simulink model "bh_motor_and_full_mech_system"  (R2017a)
settings: Solver=ode15s  StartTime=0.0  StopTime=70  FixedStep=0.001  RelTol=1e-7  EnableMultiTasking=on
undefined symbols (not defined in the file or in its folder): g, Hz, L1x, L1y, L1z, mass1, sigbuilder_block, X, Y, Z
undefined symbols (not defined in the file): Ke
libraries: simulink_extras x18, nesl_utility x13, sm_lib x13, fl_lib x12, simulink x4, elec_lib x2, discretizing x1
settings Model: Creator=bhorton  LastModifiedBy=bhorton
settings SolverCC: ZeroCrossAlgorithm=Adaptive
settings OptimizationCC: LifeSpan=inf
settings DebuggingCC: SFUnexpectedBacktrackingDiag=warning  SFNoUnconditionalDefaultTransitionDiag=warning  SFExecutionAtInitializationDiag=none
settings GRTTargetCC: TargetLangStandard=C89/C90 (ANSI)
settings ConfigComp: CovMetricSettings=dw  CovHtmlReporting=on  CovSaveCumulativeToWorkspaceVar=on  CovSaveSingleToWorkspaceVar=on  CovExternalEMLEnable=off
settings SimscapeCC: SimscapeLogDataHistory=10000  SelectedTab=Simscape Multibody
settings ExplorerConfigSet: InternalSimMechanicsExplorerSettings="<ExplorerConfiguration><canonicalview>default</canonicalview><AnimationSetting><BasePlaybackSpeed>2</BasePlaybackSpeed><PlaybackSpeedFactor>1.0</PlaybackSpeedFactor></AnimationSetting><TilePanel><TileInfo><Tiles Columns=\"1\" Count=\"1\" Rows=\"1\"><Column Left=\"2\" Weight=\"1\"/><Column Left=\"820\"/><Row Top=\"2\" Weight=\"1\"/><Row Top=\"545\"/><Tile Height=\"1\" Width=\"1\" X=\"0\" Y=\"0\"/></Tiles></TileInfo><SceneInfo><SceneViewer><BGColor><R>0.60000002384185791</R><G>0.60000002384185791</G><B>0.60000002384185791</B></BGColor><Camera><DoPerspective>off</DoPerspective><Position><X>0.3018347345439823</X><Y>0.024415264242792611</Y><Z>0.21433472519445274</Z></Position><Center><X>0.024999999062628675</X><Y>0.30124999972414623</Y><Z>-0.062500010286905439</Z></Center><Up><X>-0.40824829046386751</X><Y>0.40824829046386751</Y><Z>0.81649658092772159</Z></Up><ViewLimDist>1</ViewLimDist><YLim>0.27384785473346712</YLim><XLim>0.4148743716842227</XLim></Camera></SceneViewer></SceneInfo></TilePanel><MechEditorPanel><Cameras/><GfxPanelCameraMap/></MechEditorPanel></ExplorerConfiguration>"

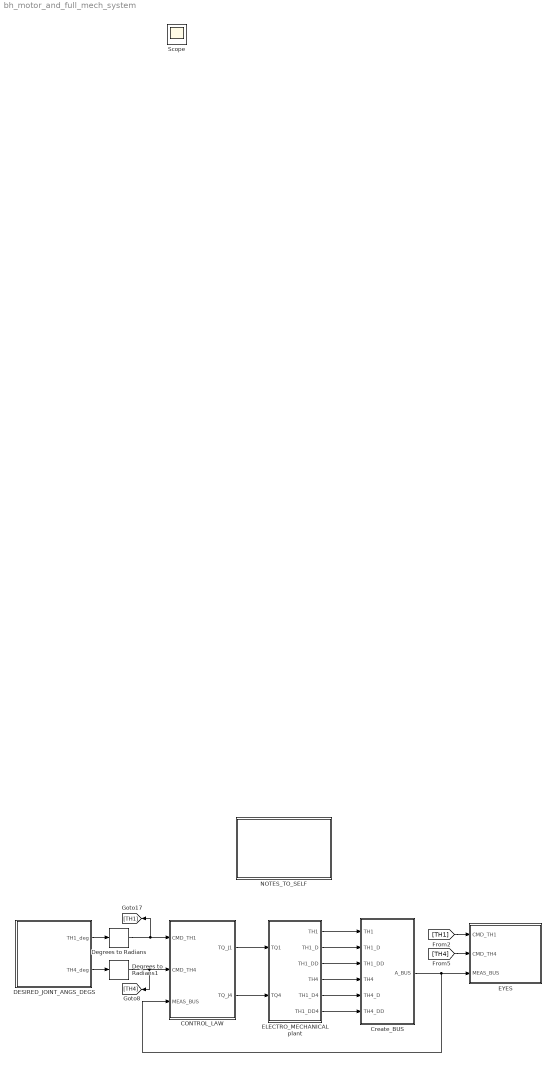
== system bh_motor_and_full_mech_system ==
  CONTROL_LAW : Subsystem
  Create_BUS : Subsystem
  DESIRED_JOINT_ANGS_DEGS : Subsystem  Tag=STV Subsys  LoadFcn=sigbuilder_block('load');  StartFcn=sigbuilder_block('start');  StopFcn=sigbuilder_block('stop');  ClipboardFcn=sigbuilder_block('clipboard');  mask(Sigbuilder block){tuvar=[0:10]}
      mask help: Simulink:masks:SigbuilderBlock_MD
      mask init:
      | if ~strcmp(get_param(bdroot(gcbh),'SimulationStatus'),'stopped') tuvar = sigbuilder_block('maskInit'); end
      settings: CopyFcn=sigbuilder_block('copy');  DeleteFcn=sigbuilder_block('delete');  ModelCloseFcn=sigbuilder_block('modelClose');  PreSaveFcn=sigbuilder_block('preSave');  PauseFcn=sigbuilder_block('pause');  ContinueFcn=sigbuilder_block('continue');  NameChangeFcn=sigbuilder_block('namechange');  OpenFcn=sigbuilder_block('open',[6 30 1428 681.75 ]);  CloseFcn=sigbuilder_block('close');
      mask Display: plot(0, 0, 100, 100,[2, 2, 32, 32, 2], [68, 8, 8, 68, 68],[32, 2], [38, 38], [32, 19, 2],[53, 60, 44], [32, 17, 17, 2],[16, 16, 31, 31]);txt = getActiveGroup(gcbh);text(2, 100, txt,'verticalAlignment', 'top');
  Degrees to Radians : simulink_extras/Transformations/Degrees to Radians
  Degrees to Radians1 : simulink_extras/Transformations/Degrees to Radians
  ELECTRO_MECHANICAL plant : Subsystem
  EYES : Subsystem
  NOTES_TO_SELF : Subsystem
  Scope : Scope
  wires:
  DESIRED_JOINT_ANGS_DEGS/1(TH1_deg) -> Degrees to Radians/1
  Degrees to Radians/1 -> CONTROL_LAW/1(CMD_TH1), [TH1]
  Degrees to Radians1/1 -> CONTROL_LAW/2(CMD_TH4), [TH4]
  DESIRED_JOINT_ANGS_DEGS/2(TH4_deg) -> Degrees to Radians1/1
  CONTROL_LAW/1(TQ_J1) -> ELECTRO_MECHANICAL plant/1(TQ1)
  CONTROL_LAW/2(TQ_J4) -> ELECTRO_MECHANICAL plant/2(TQ4)
  [TH4] -> EYES/2(CMD_TH4)
  Create_BUS/1(A_BUS) -> EYES/3(MEAS_BUS), CONTROL_LAW/3(MEAS_BUS)
  [TH1] -> EYES/1(CMD_TH1)
  ELECTRO_MECHANICAL plant/1(TH1) -> Create_BUS/1(TH1)
  ELECTRO_MECHANICAL plant/2(TH1_D) -> Create_BUS/2(TH1_D)
  ELECTRO_MECHANICAL plant/3(TH1_DD) -> Create_BUS/3(TH1_DD)
  ELECTRO_MECHANICAL plant/4(TH4) -> Create_BUS/4(TH4)
  ELECTRO_MECHANICAL plant/5(TH1_D4) -> Create_BUS/5(TH4_D)
  ELECTRO_MECHANICAL plant/6(TH1_DD4) -> Create_BUS/6(TH4_DD)

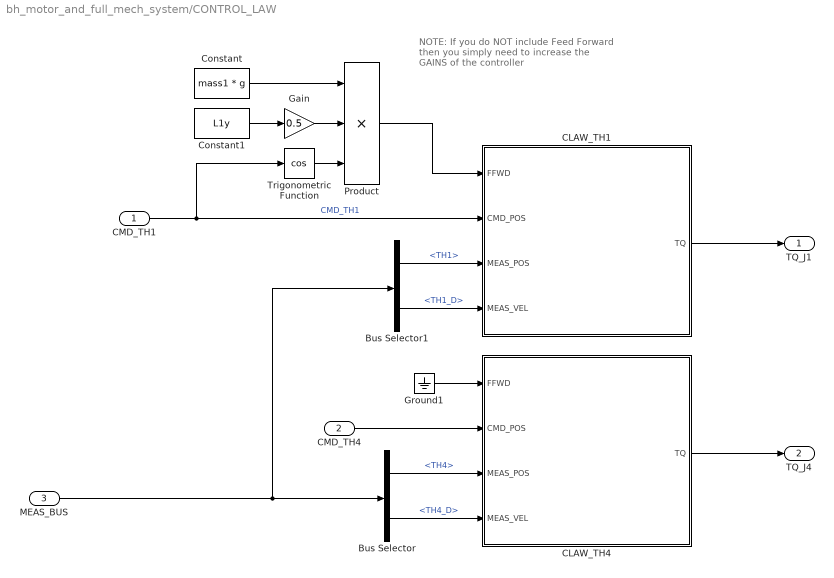
== system bh_motor_and_full_mech_system/CONTROL_LAW ==
  note: NOTE:
      | If you do NOT include Feed Forward
      | then you simply need to increase the GAINS of the controller
  CMD_TH1 : Inport
  CMD_TH4 : Inport  Port=2
  MEAS_BUS : Inport  Port=3
  Bus Selector : BusSelector  OutputSignals=TH4,TH4_D
  Bus Selector1 : BusSelector  OutputSignals=TH1,TH1_D
  CLAW_TH1 : Subsystem
  CLAW_TH4 : Subsystem
  Constant : Constant  Value=mass1 * g
  Constant1 : Constant  Value=L1y
  Gain : Gain  Gain=0.5
  Ground1 : Ground
  Product : Product  Inputs=3
  Trigonometric Function : Trigonometry  Operator=cos
  TQ_J1 : Outport
  TQ_J4 : Outport  Port=2
  wires:
  MEAS_BUS/1 -> Bus Selector1/1, Bus Selector/1
  CMD_TH4/1 -> CLAW_TH4/2(CMD_POS)
  Bus Selector/2 -> CLAW_TH4/4(MEAS_VEL)  "<TH4_D>"
  Bus Selector/1 -> CLAW_TH4/3(MEAS_POS)  "<TH4>"
  Bus Selector1/1 -> CLAW_TH1/3(MEAS_POS)  "<TH1>"
  Bus Selector1/2 -> CLAW_TH1/4(MEAS_VEL)  "<TH1_D>"
  Ground1/1 -> CLAW_TH4/1(FFWD)
  CMD_TH1/1 -> CLAW_TH1/2(CMD_POS), Trigonometric Function/1  "CMD_TH1"
  Constant/1 -> Product/1
  Constant1/1 -> Gain/1
  Product/1 -> CLAW_TH1/1(FFWD)
  Gain/1 -> Product/2
  Trigonometric Function/1 -> Product/3
  CLAW_TH1/1(TQ) -> TQ_J1/1
  CLAW_TH4/1(TQ) -> TQ_J4/1

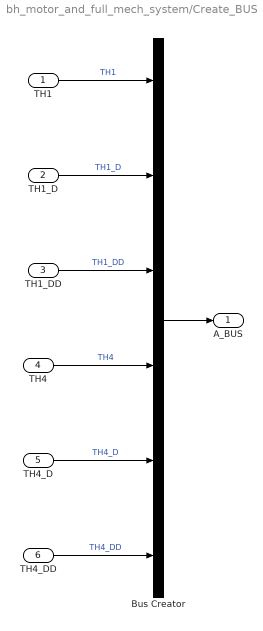
== system bh_motor_and_full_mech_system/Create_BUS ==
  TH1 : Inport
  TH1_D : Inport  Port=2
  TH1_DD : Inport  Port=3
  TH4 : Inport  Port=4
  TH4_D : Inport  Port=5
  TH4_DD : Inport  Port=6
  Bus Creator : BusCreator  Inputs=6
  A_BUS : Outport
  wires:
  TH1_DD/1 -> Bus Creator/3  "TH1_DD"
  TH1_D/1 -> Bus Creator/2  "TH1_D"
  TH1/1 -> Bus Creator/1  "TH1"
  Bus Creator/1 -> A_BUS/1
  TH4_DD/1 -> Bus Creator/6  "TH4_DD"
  TH4_D/1 -> Bus Creator/5  "TH4_D"
  TH4/1 -> Bus Creator/4  "TH4"

== system bh_motor_and_full_mech_system/DESIRED_JOINT_ANGS_DEGS ==
  Demux : Demux  Tag=STV Demux  Outputs=2
  FromWs : FromWorkspace  Tag=STV FromWs  VariableName=tuvar  SampleTime=0
      SigBuilderData=|
      | common.afterFinalStr = 'Extrapolate'
      | common.sampleTime = 0
      | dataSet(1).timeRange = [0 60]
      | dataSet(1).name = 'SCENARIO_A_JUST_TH1'
      | dataSet(2).timeRange = [0 60]
      | dataSet(2).name = 'SCENARIO_B_JUST_TH4'
      | dataSet(3).timeRange = [0 60]
      | dataSet(3).name = 'SCENARIO_C_TH1_and_TH4'
      | dataSet(4).timeRange = [0 60]
      | dataSet(4).name = 'SCENARIO_D_TH1_and_TH4'
      | dataSet(5).timeRange = [0 70]
      | dataSet(5).name = 'SCENARIO_E'
      | sbobj.Groups(1).Name = 'SCENARIO_A_JUST_TH1'
      | sbobj.Groups(1).Signals(1).Name = 'TH1_deg'
      | sbobj.Groups(1).Signals(1).XData = [0 20 20 60]
      | sbobj.Groups(1).Signals(1).YData = [0 0 45 45]
      | sbobj.Groups(1).Signals(2).Name = 'TH4_deg'
      | sbobj.Groups(1).Signals(2).XData = [0 60]
      | sbobj.Groups(1).Signals(2).YData = [0 0]
      | sbobj.Groups(1).TimeRange = [0 60]
      | sbobj.Groups(2).Name = 'SCENARIO_B_JUST_TH4'
      | sbobj.Groups(2).Signals(1).Name = 'TH1_deg'
      | sbobj.Groups(2).Signals(1).XData = [0 20 60]
      | sbobj.Groups(2).Signals(1).YData = [0 0 0]
      | sbobj.Groups(2).Signals(2).Name = 'TH4_deg'
      | sbobj.Groups(2).Signals(2).XData = [0 20 20 60]
      | sbobj.Groups(2).Signals(2).YData = [0 0 45 45]
      | sbobj.Groups(2).TimeRange = [0 60]
      | sbobj.Groups(3).Name = 'SCENARIO_C_TH1_and_TH4'
      | sbobj.Groups(3).Signals(1).Name = 'TH1_deg'
      | sbobj.Groups(3).Signals(1).XData = [0 10 10 40 60]
      | sbobj.Groups(3).Signals(1).YData = [0 0 45 45 0]
      | sbobj.Groups(3).Signals(2).Name = 'TH4_deg'
      | sbobj.Groups(3).Signals(2).XData = [0 14.95 14.95 30 60]
      | sbobj.Groups(3).Signals(2).YData = [0 0 45 45 0]
      | sbobj.Groups(3).TimeRange = [0 60]
      | sbobj.Groups(4).Name = 'SCENARIO_D_TH1_and_TH4'
      | sbobj.Groups(4).Signals(1).Name = 'TH1_deg'
      | sbobj.Groups(4).Signals(1).XData = [0 10 40 60]
      | sbobj.Groups(4).Signals(1).YData = [0 45 45 0]
      | sbobj.Groups(4).Signals(2).Name = 'TH4_deg'
      | sbobj.Groups(4).Signals(2).XData = [0 10 30 60]
      | sbobj.Groups(4).Signals(2).YData = [0 45 45 0]
      | sbobj.Groups(4).TimeRange = [0 60]
      | sbobj.Groups(5).Name = 'SCENARIO_E'
      | sbobj.Groups(5).Signals(1).Name = 'TH1_deg'
      | sbobj.Groups(5).Signals(1).XData = [0 35.15 45.4 60 70]
      | sbobj.Groups(5).Signals(1).YData = [0 0 45 -45 0]
      | sbobj.Groups(5).Signals(2).Name = 'TH4_deg'
      | sbobj.Groups(5).Signals(2).XData = [0 10 25 30 70]
      | sbobj.Groups(5).Signals(2).YData = [0 -90 90 0 0]
      | sbobj.Groups(5).TimeRange = [0 70]
  TH1_deg : Outport  Tag=STV Outport
  TH4_deg : Outport  Tag=STV Outport  Port=2
  wires:
  FromWs/1 -> Demux/1
  Demux/1 -> TH1_deg/1
  Demux/2 -> TH4_deg/1

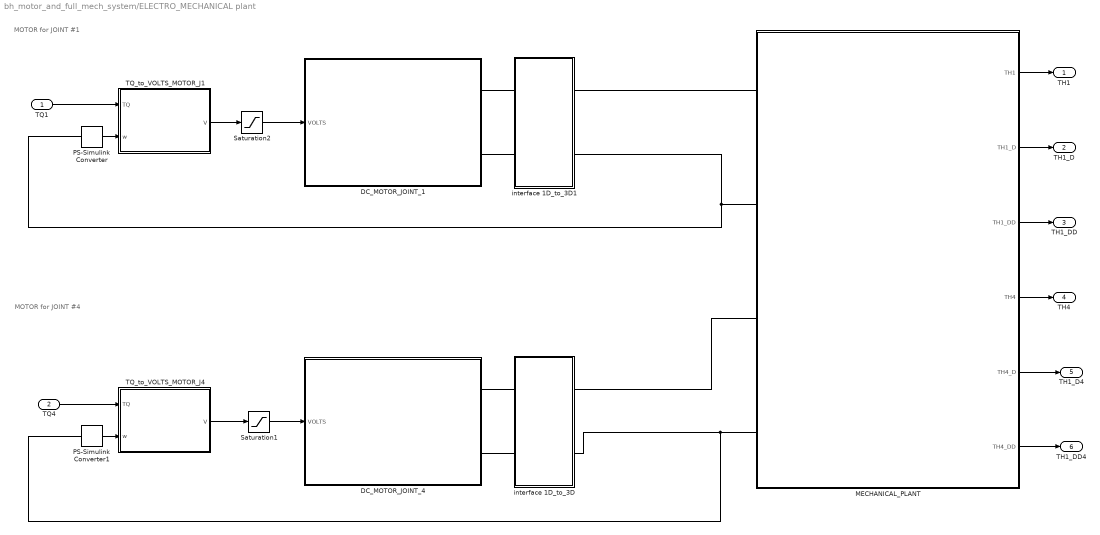
== system bh_motor_and_full_mech_system/ELECTRO_MECHANICAL plant ==
  note: MOTOR for JOINT #4
  note: MOTOR for JOINT #1
  TQ1 : Inport
  TQ4 : Inport  Port=2
  DC_MOTOR_JOINT_1 : Subsystem
      mask Display: image('bh_PIC_MOTOR.jpg');
  DC_MOTOR_JOINT_4 : Subsystem
      mask Display: image('bh_PIC_MOTOR.jpg');
  MECHANICAL_PLANT : Subsystem  VariantControl=Variant1
  PS-Simulink Converter : nesl_utility/PS-Simulink Converter  PhysicalDomain=network_engine_domain  SubClassName=ps_output  LeftPortType=input  RightPortType=output  PseudoPeriodic=off  Frequencies=[]  Unit=rad/s  AffineConversion=off
      settings: AttributesFormatString=Units = %<Unit>
  PS-Simulink Converter1 : nesl_utility/PS-Simulink Converter  PhysicalDomain=network_engine_domain  SubClassName=ps_output  LeftPortType=input  RightPortType=output  PseudoPeriodic=off  Frequencies=[]  Unit=rad/s  AffineConversion=off
      settings: AttributesFormatString=Units = %<Unit>
  Saturation1 : Saturate  UpperLimit=12  LowerLimit=-12
      settings: AttributesFormatString=|
      | Vmax = %<UpperLimit>
      | Vmin = %<LowerLimit>
  Saturation2 : Saturate  UpperLimit=12  LowerLimit=-12
      settings: AttributesFormatString=|
      | Vmax = %<UpperLimit>
      | Vmin = %<LowerLimit>
  TQ_to_VOLTS_MOTOR_J1 : Subsystem  mask(DC motor (w_IN and TQ_out)){R=5.0117, K=0.57296 *0.875, Kb=Ke, b=8.20705e-3}
      mask prompts: R "Armature resistance (ohms)"; K "Torque constant (N.m/A)"; Kb "Back Emf constant (V.sec/rad)"; b "damping value (N.m.sec/rad)"
      mask help: A DC motor model that outputs required VOLTAGE needed to deliver a specified TORQUE
      mask DialogControl Control2 Prompt: NOTE:  with SI units, the Toque constant (Ka) and Back EMF constant(Kb) are the same.
      mask DialogControl Container9 Prompt: Electrical
      mask Display: fprintf('DC motor\n(TQ_IN \n and \n V_out)');
  TQ_to_VOLTS_MOTOR_J4 : Subsystem  mask(DC motor (w_IN and TQ_out)){R=5.0117, K=0.57296 *0.875, Kb=Ke, b=8.20705e-3}
      mask prompts: R "Armature resistance (ohms)"; K "Torque constant (N.m/A)"; Kb "Back Emf constant (V.sec/rad)"; b "damping value (N.m.sec/rad)"
      mask help: A DC motor model that outputs required VOLTAGE needed to deliver a specified TORQUE
      mask DialogControl Control2 Prompt: NOTE:  with SI units, the Toque constant (Ka) and Back EMF constant(Kb) are the same.
      mask DialogControl Container9 Prompt: Electrical
      mask Display: fprintf('DC motor\n(TQ_IN \n and \n V_out)');
  interface 1D_to_3D : Subsystem
  interface 1D_to_3D1 : Subsystem
  TH1 : Outport
  TH1_D : Outport  Port=2
  TH1_DD : Outport  Port=3
  TH4 : Outport  Port=4
  TH1_D4 : Outport  Port=5
  TH1_DD4 : Outport  Port=6
  wires:
  TQ_to_VOLTS_MOTOR_J1/1(V) -> Saturation2/1
  PS-Simulink Converter/1 -> TQ_to_VOLTS_MOTOR_J1/2(w)
  TQ1/1 -> TQ_to_VOLTS_MOTOR_J1/1(TQ)
  PS-Simulink Converter1/1 -> TQ_to_VOLTS_MOTOR_J4/2(w)
  TQ4/1 -> TQ_to_VOLTS_MOTOR_J4/1(TQ)
  TQ_to_VOLTS_MOTOR_J4/1(V) -> Saturation1/1
  MECHANICAL_PLANT/1(TH1) -> TH1/1
  MECHANICAL_PLANT/2(TH1_D) -> TH1_D/1
  MECHANICAL_PLANT/3(TH1_DD) -> TH1_DD/1
  MECHANICAL_PLANT/4(TH4) -> TH4/1
  MECHANICAL_PLANT/5(TH4_D) -> TH1_D4/1
  MECHANICAL_PLANT/6(TH4_DD) -> TH1_DD4/1
  Saturation1/1 -> DC_MOTOR_JOINT_4/1(VOLTS)
  Saturation2/1 -> DC_MOTOR_JOINT_1/1(VOLTS)
  connections:
  interface 1D_to_3D/RConn1 -- MECHANICAL_PLANT/LConn3
  PS-Simulink Converter/LConn1 -- interface 1D_to_3D1/RConn2 -- MECHANICAL_PLANT/LConn2
  interface 1D_to_3D/RConn2 -- PS-Simulink Converter1/LConn1 -- MECHANICAL_PLANT/LConn4
  MECHANICAL_PLANT/LConn1 -- interface 1D_to_3D1/RConn1
  interface 1D_to_3D/LConn1 -- DC_MOTOR_JOINT_4/RConn1
  interface 1D_to_3D/LConn2 -- DC_MOTOR_JOINT_4/RConn2
  interface 1D_to_3D1/LConn1 -- DC_MOTOR_JOINT_1/RConn1
  interface 1D_to_3D1/LConn2 -- DC_MOTOR_JOINT_1/RConn2

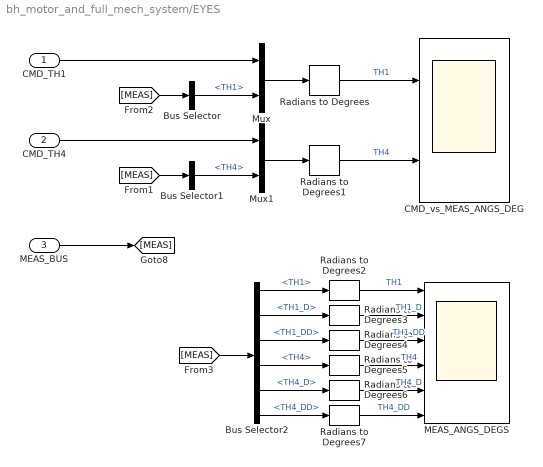
== system bh_motor_and_full_mech_system/EYES ==
  CMD_TH1 : Inport
  CMD_TH4 : Inport  Port=2
  MEAS_BUS : Inport  Port=3
  Bus Selector : BusSelector  OutputSignals=TH1
  Bus Selector1 : BusSelector  OutputSignals=TH4
  Bus Selector2 : BusSelector  OutputSignals=TH1,TH1_D,TH1_DD,TH4,TH4_D,TH4_DD
  CMD_vs_MEAS_ANGS_DEG : Scope  NumInputPorts=2
  MEAS_ANGS_DEGS : Scope  NumInputPorts=6
  Mux : Mux  Inputs=2
  Mux1 : Mux  Inputs=2
  Radians to Degrees{,1..7} (8 alike) : simulink_extras/Transformations/Radians to Degrees
  wires:
  MEAS_BUS/1 -> [MEAS]
  CMD_TH1/1 -> Mux/1
  Bus Selector/1 -> Mux/2  "<TH1>"
  [MEAS] -> Bus Selector/1
  Mux/1 -> Radians to Degrees/1
  CMD_TH4/1 -> Mux1/1
  Bus Selector1/1 -> Mux1/2  "<TH4>"
  [MEAS] -> Bus Selector1/1
  Mux1/1 -> Radians to Degrees1/1
  Radians to Degrees1/1 -> CMD_vs_MEAS_ANGS_DEG/2  "TH4"
  Radians to Degrees/1 -> CMD_vs_MEAS_ANGS_DEG/1  "TH1"
  [MEAS] -> Bus Selector2/1
  Bus Selector2/6 -> Radians to Degrees7/1  "<TH4_DD>"
  Bus Selector2/3 -> Radians to Degrees4/1  "<TH1_DD>"
  Bus Selector2/4 -> Radians to Degrees5/1  "<TH4>"
  Bus Selector2/5 -> Radians to Degrees6/1  "<TH4_D>"
  Bus Selector2/2 -> Radians to Degrees3/1  "<TH1_D>"
  Bus Selector2/1 -> Radians to Degrees2/1  "<TH1>"
  Radians to Degrees2/1 -> MEAS_ANGS_DEGS/1  "TH1"
  Radians to Degrees3/1 -> MEAS_ANGS_DEGS/2  "TH1_D"
  Radians to Degrees4/1 -> MEAS_ANGS_DEGS/3  "TH1_DD"
  Radians to Degrees5/1 -> MEAS_ANGS_DEGS/4  "TH4"
  Radians to Degrees6/1 -> MEAS_ANGS_DEGS/5  "TH4_D"
  Radians to Degrees7/1 -> MEAS_ANGS_DEGS/6  "TH4_DD"

== system bh_motor_and_full_mech_system/NOTES_TO_SELF ==
  note: NOTES to self:
      | Had to enable these:

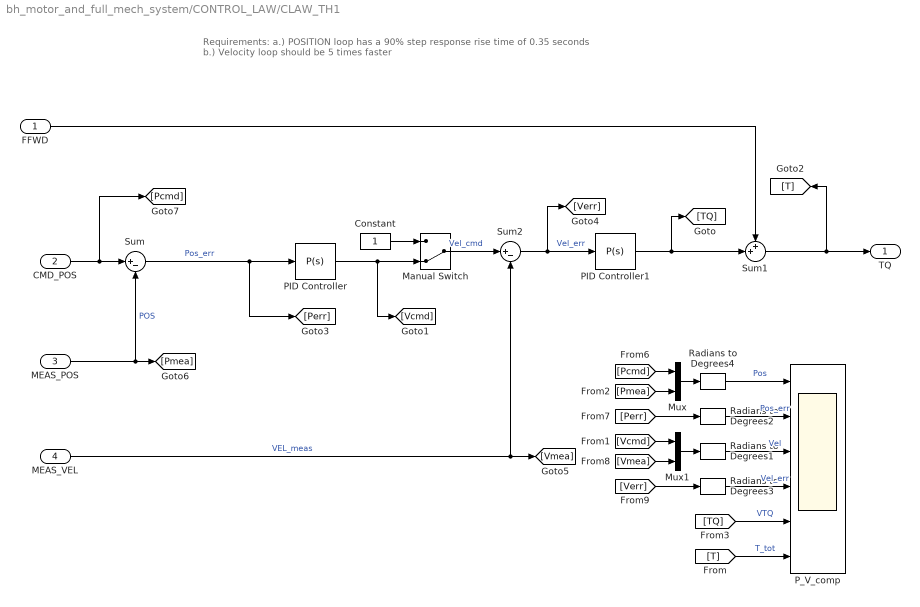
== system bh_motor_and_full_mech_system/CONTROL_LAW/CLAW_TH1 ==
  note: Requirements:
      | a.) POSITION loop has a 90% step response
      | rise time of 0.35 seconds
      |
      | b.) Velocity loop should be 5 times faster
  FFWD : Inport
  CMD_POS : Inport  Port=2
  MEAS_POS : Inport  Port=3
  MEAS_VEL : Inport  Port=4
  Constant : Constant
  Manual Switch : ManualSwitch  CurrentSetting=0
  Mux : Mux  Inputs=2
  Mux1 : Mux  Inputs=2
  PID Controller : simulink/Continuous/PID Controller  Controller=P  TimeDomain=Continuous-time  SampleTime=-1  IntegratorMethod=Forward Euler  FilterMethod=Forward Euler  Form=Parallel  UseFilter=on  ControllerParametersSource=internal  P=5.58549433794614  I=0  D=0  N=100  InitialConditionSource=internal  InitialConditionForIntegrator=0  InitialConditionForFilter=0  ExternalReset=none  LimitOutput=off  UpperSaturationLimit=inf  LowerSaturationLimit=-inf  LinearizeAsGain=on  AntiWindupMode=none  Kb=1  TrackingMode=off  Kt=1  PParamMin=[]  PParamMax=[]  IParamMin=[]  IParamMax=[]  DParamMin=[]  DParamMax=[]  NParamMin=[]  NParamMax=[]  KbParamMin=[]  KbParamMax=[]  KtParamMin=[]  KtParamMax=[]  POutMin=[]  POutMax=[]  IOutMin=[]  IOutMax=[]  DOutMin=[]  DOutMax=[]  NOutMin=[]  NOutMax=[]  KbOutMin=[]  KbOutMax=[]  KtOutMin=[]  KtOutMax=[]  IntegratorOutMin=[]  IntegratorOutMax=[]  FilterOutMin=[]  FilterOutMax=[]  SumOutMin=[]  SumOutMax=[]  SumI1OutMin=[]  SumI1OutMax=[]  SumI2OutMin=[]  SumI2OutMax=[]  SumI3OutMin=[]  SumI3OutMax=[]  SumDOutMin=[]  SumDOutMax=[]  SaturationOutMin=[]  SaturationOutMax=[]  IntegratorContinuousStateAttributes=''  IntegratorStateMustResolveToSignalObject=off  IntegratorRTWStateStorageClass=Auto  FilterContinuousStateAttributes=''  FilterStateMustResolveToSignalObject=off  FilterRTWStateStorageClass=Auto  DifferentiatorICPrevScaledInput=0  DifferentiatorOutMin=[]  DifferentiatorOutMax=[]  InitialConditionSetting=State (most efficient)
  PID Controller1 : simulink/Continuous/PID Controller  Controller=P  TimeDomain=Continuous-time  SampleTime=-1  IntegratorMethod=Forward Euler  FilterMethod=Forward Euler  Form=Parallel  UseFilter=on  ControllerParametersSource=internal  P=1  I=1  D=0  N=100  InitialConditionSource=internal  InitialConditionForIntegrator=0  InitialConditionForFilter=0  ExternalReset=none  LimitOutput=off  UpperSaturationLimit=inf  LowerSaturationLimit=-inf  LinearizeAsGain=on  AntiWindupMode=none  Kb=1  TrackingMode=off  Kt=1  PParamMin=[]  PParamMax=[]  IParamMin=[]  IParamMax=[]  DParamMin=[]  DParamMax=[]  NParamMin=[]  NParamMax=[]  KbParamMin=[]  KbParamMax=[]  KtParamMin=[]  KtParamMax=[]  POutMin=[]  POutMax=[]  IOutMin=[]  IOutMax=[]  DOutMin=[]  DOutMax=[]  NOutMin=[]  NOutMax=[]  KbOutMin=[]  KbOutMax=[]  KtOutMin=[]  KtOutMax=[]  IntegratorOutMin=[]  IntegratorOutMax=[]  FilterOutMin=[]  FilterOutMax=[]  SumOutMin=[]  SumOutMax=[]  SumI1OutMin=[]  SumI1OutMax=[]  SumI2OutMin=[]  SumI2OutMax=[]  SumI3OutMin=[]  SumI3OutMax=[]  SumDOutMin=[]  SumDOutMax=[]  SaturationOutMin=[]  SaturationOutMax=[]  IntegratorContinuousStateAttributes=''  IntegratorStateMustResolveToSignalObject=off  IntegratorRTWStateStorageClass=Auto  FilterContinuousStateAttributes=''  FilterStateMustResolveToSignalObject=off  FilterRTWStateStorageClass=Auto  DifferentiatorICPrevScaledInput=0  DifferentiatorOutMin=[]  DifferentiatorOutMax=[]  InitialConditionSetting=State (most efficient)
  P_V_comp : Scope  NumInputPorts=6
  Radians to Degrees{1..4} (4 alike) : simulink_extras/Transformations/Radians to Degrees
  Sum : Sum  Inputs=|+-
  Sum1 : Sum  Inputs=++|
  Sum2 : Sum  Inputs=|+-
  TQ : Outport
  wires:
  FFWD/1 -> Sum1/1
  CMD_POS/1 -> [Pcmd], Sum/1
  MEAS_VEL/1 -> [Vmea], Sum2/2  "VEL_meas"
  MEAS_POS/1 -> [Pmea], Sum/2  "POS"
  Sum2/1 -> PID Controller1/1, [Verr]  "Vel_err"
  Manual Switch/1 -> Sum2/1  "Vel_cmd"
  Constant/1 -> Manual Switch/1
  Sum/1 -> PID Controller/1, [Perr]  "Pos_err"
  PID Controller/1 -> Manual Switch/2, [Vcmd]
  Sum1/1 -> TQ/1, [T]
  Mux/1 -> Radians to Degrees4/1
  [Pcmd] -> Mux/1
  [Pmea] -> Mux/2
  Mux1/1 -> Radians to Degrees1/1
  [Vcmd] -> Mux1/1
  [Vmea] -> Mux1/2
  [Verr] -> Radians to Degrees3/1
  [Perr] -> Radians to Degrees2/1
  Radians to Degrees3/1 -> P_V_comp/4  "Vel_err"
  Radians to Degrees2/1 -> P_V_comp/2  "Pos_err"
  Radians to Degrees1/1 -> P_V_comp/3  "Vel"
  Radians to Degrees4/1 -> P_V_comp/1  "Pos"
  [TQ] -> P_V_comp/5  "VTQ"
  [T] -> P_V_comp/6  "T_tot"
  PID Controller1/1 -> Sum1/2, [TQ]

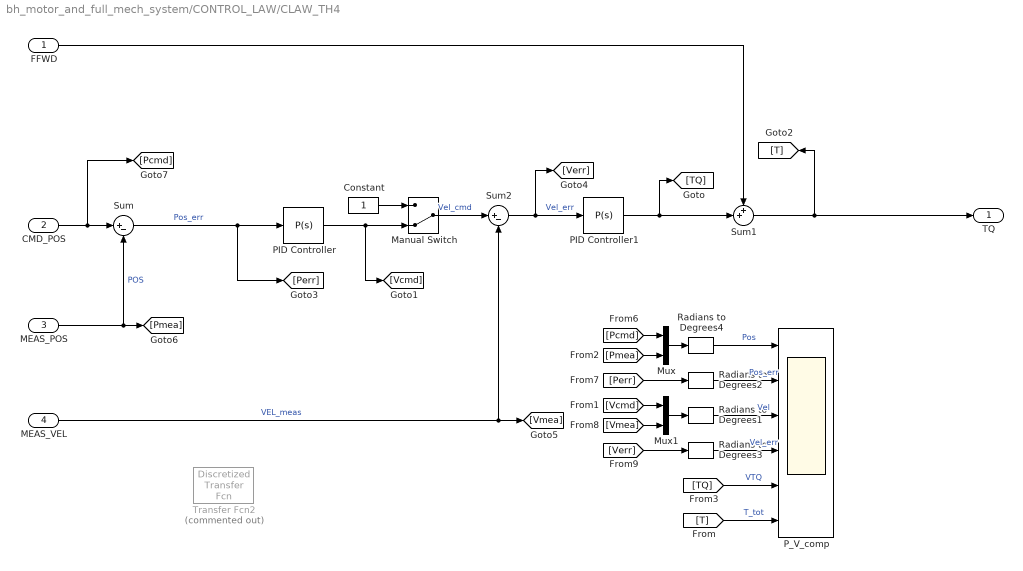
== system bh_motor_and_full_mech_system/CONTROL_LAW/CLAW_TH4 ==
  FFWD : Inport
  CMD_POS : Inport  Port=2
  MEAS_POS : Inport  Port=3
  MEAS_VEL : Inport  Port=4
  Constant : Constant
  Manual Switch : ManualSwitch  CurrentSetting=0
  Mux : Mux  Inputs=2
  Mux1 : Mux  Inputs=2
  PID Controller : simulink/Continuous/PID Controller  Controller=P  TimeDomain=Continuous-time  SampleTime=-1  IntegratorMethod=Forward Euler  FilterMethod=Forward Euler  Form=Parallel  UseFilter=on  ControllerParametersSource=internal  P=5.58549433794614  I=1  D=0  N=100  InitialConditionSource=internal  InitialConditionForIntegrator=0  InitialConditionForFilter=0  ExternalReset=none  LimitOutput=off  UpperSaturationLimit=inf  LowerSaturationLimit=-inf  LinearizeAsGain=on  AntiWindupMode=none  Kb=1  TrackingMode=off  Kt=1  PParamMin=[]  PParamMax=[]  IParamMin=[]  IParamMax=[]  DParamMin=[]  DParamMax=[]  NParamMin=[]  NParamMax=[]  KbParamMin=[]  KbParamMax=[]  KtParamMin=[]  KtParamMax=[]  POutMin=[]  POutMax=[]  IOutMin=[]  IOutMax=[]  DOutMin=[]  DOutMax=[]  NOutMin=[]  NOutMax=[]  KbOutMin=[]  KbOutMax=[]  KtOutMin=[]  KtOutMax=[]  IntegratorOutMin=[]  IntegratorOutMax=[]  FilterOutMin=[]  FilterOutMax=[]  SumOutMin=[]  SumOutMax=[]  SumI1OutMin=[]  SumI1OutMax=[]  SumI2OutMin=[]  SumI2OutMax=[]  SumI3OutMin=[]  SumI3OutMax=[]  SumDOutMin=[]  SumDOutMax=[]  SaturationOutMin=[]  SaturationOutMax=[]  IntegratorContinuousStateAttributes=''  IntegratorStateMustResolveToSignalObject=off  IntegratorRTWStateStorageClass=Auto  FilterContinuousStateAttributes=''  FilterStateMustResolveToSignalObject=off  FilterRTWStateStorageClass=Auto  DifferentiatorICPrevScaledInput=0  DifferentiatorOutMin=[]  DifferentiatorOutMax=[]  InitialConditionSetting=State (most efficient)
  PID Controller1 : simulink/Continuous/PID Controller  Controller=P  TimeDomain=Continuous-time  SampleTime=-1  IntegratorMethod=Forward Euler  FilterMethod=Forward Euler  Form=Parallel  UseFilter=on  ControllerParametersSource=internal  P=1  I=1  D=0  N=100  InitialConditionSource=internal  InitialConditionForIntegrator=0  InitialConditionForFilter=0  ExternalReset=none  LimitOutput=off  UpperSaturationLimit=inf  LowerSaturationLimit=-inf  LinearizeAsGain=on  AntiWindupMode=none  Kb=1  TrackingMode=off  Kt=1  PParamMin=[]  PParamMax=[]  IParamMin=[]  IParamMax=[]  DParamMin=[]  DParamMax=[]  NParamMin=[]  NParamMax=[]  KbParamMin=[]  KbParamMax=[]  KtParamMin=[]  KtParamMax=[]  POutMin=[]  POutMax=[]  IOutMin=[]  IOutMax=[]  DOutMin=[]  DOutMax=[]  NOutMin=[]  NOutMax=[]  KbOutMin=[]  KbOutMax=[]  KtOutMin=[]  KtOutMax=[]  IntegratorOutMin=[]  IntegratorOutMax=[]  FilterOutMin=[]  FilterOutMax=[]  SumOutMin=[]  SumOutMax=[]  SumI1OutMin=[]  SumI1OutMax=[]  SumI2OutMin=[]  SumI2OutMax=[]  SumI3OutMin=[]  SumI3OutMax=[]  SumDOutMin=[]  SumDOutMax=[]  SaturationOutMin=[]  SaturationOutMax=[]  IntegratorContinuousStateAttributes=''  IntegratorStateMustResolveToSignalObject=off  IntegratorRTWStateStorageClass=Auto  FilterContinuousStateAttributes=''  FilterStateMustResolveToSignalObject=off  FilterRTWStateStorageClass=Auto  DifferentiatorICPrevScaledInput=0  DifferentiatorOutMin=[]  DifferentiatorOutMax=[]  InitialConditionSetting=State (most efficient)
  P_V_comp : Scope  NumInputPorts=6
  Radians to Degrees{1..4} (4 alike) : simulink_extras/Transformations/Radians to Degrees
  Sum : Sum  Inputs=|+-
  Sum1 : Sum  Inputs=++|
  Sum2 : Sum  Inputs=|+-
  Transfer Fcn2 : discretizing/Discretized Transfer Fcn  Commented=on  Numerator=[100]  Denominator=[1 100]  AbsTol=auto  SampleTime=0.001  method=tustin  Wc=1
  TQ : Outport
  wires:
  FFWD/1 -> Sum1/1
  CMD_POS/1 -> [Pcmd], Sum/1
  MEAS_VEL/1 -> [Vmea], Sum2/2  "VEL_meas"
  MEAS_POS/1 -> [Pmea], Sum/2  "POS"
  Sum2/1 -> PID Controller1/1, [Verr]  "Vel_err"
  Manual Switch/1 -> Sum2/1  "Vel_cmd"
  Constant/1 -> Manual Switch/1
  Sum/1 -> PID Controller/1, [Perr]  "Pos_err"
  PID Controller/1 -> Manual Switch/2, [Vcmd]
  Sum1/1 -> TQ/1, [T]
  Mux/1 -> Radians to Degrees4/1
  [Pcmd] -> Mux/1
  [Pmea] -> Mux/2
  Mux1/1 -> Radians to Degrees1/1
  [Vcmd] -> Mux1/1
  [Vmea] -> Mux1/2
  [Verr] -> Radians to Degrees3/1
  [Perr] -> Radians to Degrees2/1
  Radians to Degrees3/1 -> P_V_comp/4  "Vel_err"
  Radians to Degrees2/1 -> P_V_comp/2  "Pos_err"
  Radians to Degrees1/1 -> P_V_comp/3  "Vel"
  Radians to Degrees4/1 -> P_V_comp/1  "Pos"
  [TQ] -> P_V_comp/5  "VTQ"
  [T] -> P_V_comp/6  "T_tot"
  PID Controller1/1 -> Sum1/2, [TQ]

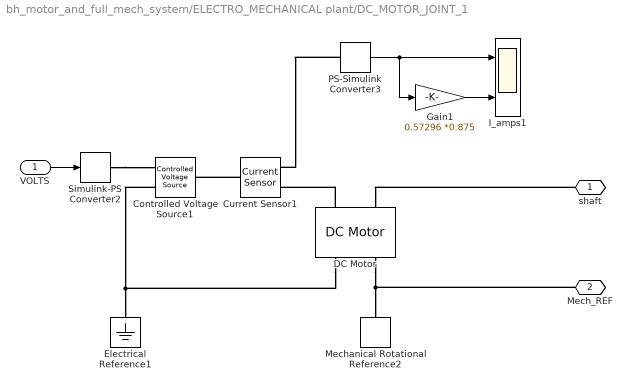
== system bh_motor_and_full_mech_system/ELECTRO_MECHANICAL plant/DC_MOTOR_JOINT_1 ==
  VOLTS : Inport
  Controlled Voltage Source1 : fl_lib/Electrical/Electrical Sources/Controlled Voltage Source
  Current Sensor1 : fl_lib/Electrical/Electrical Sensors/Current Sensor
  DC Motor : elec_lib/Actuators & Drivers/Rotational Actuators/DC Motor  parameterization=2  Ra=2 Ohm  La=1e-4 H  emf_or_torque=2  Kv=7.2e-5 V/rpm  Ki=0.0083 N*m/A  T_stall=1.2 N*m  w_max=200 rpm  w_rated=1.5e+4 rpm  P_rated=0.08 W  V_rated=12 V  J=4.5e-5 kg*m^2  lam_param=2  lam=0.7e-5 N*m/(rad/s)  i_noload=300 mA  V_i_noload=12 V  speed0=0 rpm  alpha=0.00393 1/K  Tmeas=25 C  thermal_mass=100 J/K  initial_temperature=25 C
  Electrical Reference1 : fl_lib/Electrical/Electrical Elements/Electrical Reference
  Gain1 : Gain  Gain=0.57296 *0.875
  I_amps1 : Scope  NumInputPorts=2
  Mechanical Rotational Reference2 : fl_lib/Mechanical/Rotational Elements/Mechanical Rotational Reference
  PS-Simulink Converter3 : nesl_utility/PS-Simulink Converter  PhysicalDomain=network_engine_domain  SubClassName=ps_output  LeftPortType=input  RightPortType=output  PseudoPeriodic=off  Frequencies=[]  Unit=A  AffineConversion=off
  Simulink-PS Converter2 : nesl_utility/Simulink-PS Converter  PhysicalDomain=network_engine_domain  SubClassName=ps_input  LeftPortType=input  RightPortType=output  PseudoPeriodic=off  Frequencies=[]  NoiseDistribution=none  NoiseParameters=[]  Unit=V  AffineConversion=off  FilteringAndDerivatives=filter  SimscapeFilterOrder=1  InputFilterTimeConstant=0.001  UdotUserProvided=1
  shaft : PMIOPort  Port=1  Side=Right
  Mech_REF : PMIOPort  Port=2  Side=Right
  wires:
  Gain1/1 -> I_amps1/2
  VOLTS/1 -> Simulink-PS Converter2/1
  PS-Simulink Converter3/1 -> Gain1/1, I_amps1/1
  connections:
  DC Motor/LConn1 -- Current Sensor1/RConn2
  DC Motor/RConn2 -- Mechanical Rotational Reference2/LConn1 -- Mech_REF/RConn1
  Current Sensor1/LConn1 -- Controlled Voltage Source1/LConn1
  Simulink-PS Converter2/RConn1 -- Controlled Voltage Source1/RConn1
  shaft/RConn1 -- DC Motor/LConn2
  Controlled Voltage Source1/RConn2 -- DC Motor/RConn1 -- Electrical Reference1/LConn1
  PS-Simulink Converter3/LConn1 -- Current Sensor1/RConn1

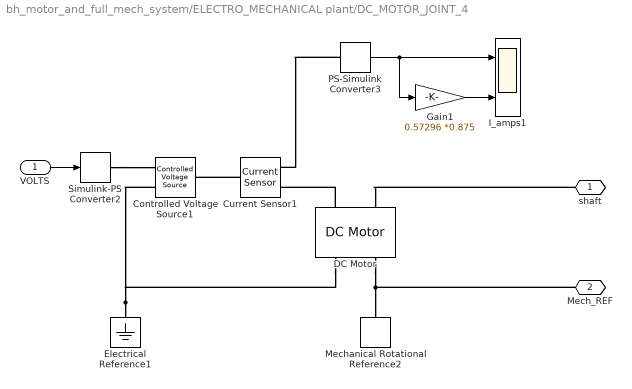
== system bh_motor_and_full_mech_system/ELECTRO_MECHANICAL plant/DC_MOTOR_JOINT_4 ==
  VOLTS : Inport
  Controlled Voltage Source1 : fl_lib/Electrical/Electrical Sources/Controlled Voltage Source
  Current Sensor1 : fl_lib/Electrical/Electrical Sensors/Current Sensor
  DC Motor : elec_lib/Actuators & Drivers/Rotational Actuators/DC Motor  parameterization=2  Ra=2 Ohm  La=1e-4 H  emf_or_torque=2  Kv=7.2e-5 V/rpm  Ki=0.0083 N*m/A  T_stall=1.2 N*m  w_max=200 rpm  w_rated=1.5e+4 rpm  P_rated=0.08 W  V_rated=12 V  J=4.5e-5 kg*m^2  lam_param=2  lam=0.7e-5 N*m/(rad/s)  i_noload=300 mA  V_i_noload=12 V  speed0=0 rpm  alpha=0.00393 1/K  Tmeas=25 C  thermal_mass=100 J/K  initial_temperature=25 C
  Electrical Reference1 : fl_lib/Electrical/Electrical Elements/Electrical Reference
  Gain1 : Gain  Gain=0.57296 *0.875
  I_amps1 : Scope  NumInputPorts=2
  Mechanical Rotational Reference2 : fl_lib/Mechanical/Rotational Elements/Mechanical Rotational Reference
  PS-Simulink Converter3 : nesl_utility/PS-Simulink Converter  PhysicalDomain=network_engine_domain  SubClassName=ps_output  LeftPortType=input  RightPortType=output  PseudoPeriodic=off  Frequencies=[]  Unit=A  AffineConversion=off
  Simulink-PS Converter2 : nesl_utility/Simulink-PS Converter  PhysicalDomain=network_engine_domain  SubClassName=ps_input  LeftPortType=input  RightPortType=output  PseudoPeriodic=off  Frequencies=[]  NoiseDistribution=none  NoiseParameters=[]  Unit=V  AffineConversion=off  FilteringAndDerivatives=filter  SimscapeFilterOrder=1  InputFilterTimeConstant=0.001  UdotUserProvided=1
  shaft : PMIOPort  Port=1  Side=Right
  Mech_REF : PMIOPort  Port=2  Side=Right
  wires:
  Gain1/1 -> I_amps1/2
  VOLTS/1 -> Simulink-PS Converter2/1
  PS-Simulink Converter3/1 -> Gain1/1, I_amps1/1
  connections:
  DC Motor/LConn1 -- Current Sensor1/RConn2
  DC Motor/RConn2 -- Mech_REF/RConn1 -- Mechanical Rotational Reference2/LConn1
  Current Sensor1/LConn1 -- Controlled Voltage Source1/LConn1
  Simulink-PS Converter2/RConn1 -- Controlled Voltage Source1/RConn1
  shaft/RConn1 -- DC Motor/LConn2
  Electrical Reference1/LConn1 -- Controlled Voltage Source1/RConn2 -- DC Motor/RConn1
  PS-Simulink Converter3/LConn1 -- Current Sensor1/RConn1

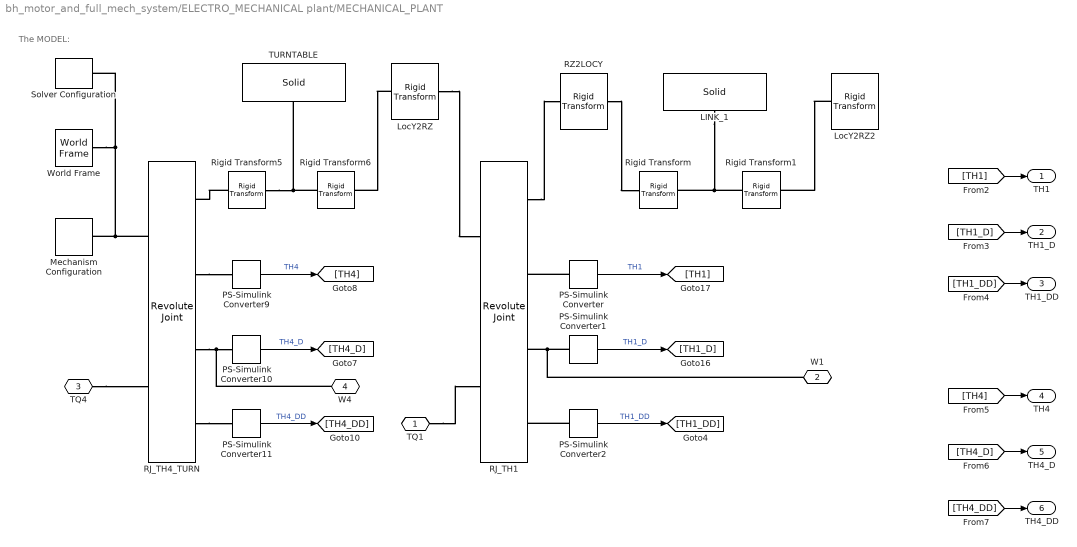
== system bh_motor_and_full_mech_system/ELECTRO_MECHANICAL plant/MECHANICAL_PLANT ==
  note: The MODEL:
  LINK_1 : sm_lib/Body Elements/Solid  InertiaType=CalculateFromGeometry  Mass=1  MassUnits=kg  CenterOfMass=[0 0 0]  CenterOfMassUnits=m  MomentsOfInertia=[1 1 1]  MomentsOfInertiaUnits=kg*m^2  ProductsOfInertia=[0 0 0]  ProductsOfInertiaUnits=kg*m^2  DensityBased=on  Density=density  DensityUnits=kg/(m^3)  DoExposeReferenceFrame=on  SerializedFrames=<Frames/>  GraphicType=FromGeometry  MarkerShape=Sphere  MarkerSize=10  GraphicVisPropType=SimpleVisualProperties  GraphicDiffuseColor=[0.2 0.2 1.0]  GraphicSpecularColor=[0.5 0.5 0.5 1.0]  GraphicAmbientColor=[0.15 0.15 0.15 1.0]  GraphicEmissiveColor=[0.0 0.0 0.0 1.0]  GraphicShininess=75  GraphicOpacity=1.0  GeometryShape=Brick  RectangleSize=[1 1]  RectangleSizeUnits=m  BrickDimensions=[L1x, L1y, L1z ]  BrickDimensionUnits=m  CylinderRadius=1  CylinderRadiusUnits=m  CylinderLength=1  CylinderLengthUnits=m  SphereRadius=1  SphereRadiusUnits=m  EllipsoidRadii=[1 1 1]  EllipsoidRadiiUnits=m  ExtrusionCrossSection=[1 1; -1 1; -1 -1; 1 -1]  ExtrusionCrossSectionUnits=m  ExtrusionLength=1  ExtrusionLengthUnits=m  PolygonNumSides=3  PolygonOuterRadius=1  PolygonOuterRadiusUnits=m  ExtGeomFileType=STEP  ExtGeomFileUnits=m  RevolutionCrossSection=[1 1; 1 -1; 2 -1; 2 1]  RevolutionCrossSectionUnits=m  RevolutionExtent=Full  RevolutionAngle=180  RevolutionAngleUnits=deg
  LocY2RZ : sm_lib/Frames and Transforms/Rigid Transform  TranslationMethod=None  TranslationStandardOffset=Hz/2  TranslationLengthUnit=m  TranslationStandardAxis=+Z  TranslationCartesianOffset=[0 0 0]  TranslationROffset=0  TranslationROffsetUnits=m  TranslationZOffset=0  TranslationZOffsetUnits=m  TranslationThetaOffset=0  TranslationThetaOffsetUnits=deg  RotationMethod=AlignedAxes  RotationAngleUnits=deg  RotationStandardAxis=+Z  RotationAngle=0.0  RotationArbitraryAxis=[0 0 1]  FollAlignAxisA=+X  BaseAlignAxisA=+Y  FollAlignAxisB=+Y  BaseAlignAxisB=+Z  RotationSequenceAxes=FollowerAxes  RotationSequence=XYX  RotationSequenceAngles=[0 0 0]  RotationSequenceAnglesUnits=deg  RotationMatrix=[1 0 0; 0 1 0; 0 0 1]
  LocY2RZ2 : sm_lib/Frames and Transforms/Rigid Transform  TranslationMethod=None  TranslationStandardOffset=Hz/2  TranslationLengthUnit=m  TranslationStandardAxis=+Z  TranslationCartesianOffset=[0 0 0]  TranslationROffset=0  TranslationROffsetUnits=m  TranslationZOffset=0  TranslationZOffsetUnits=m  TranslationThetaOffset=0  TranslationThetaOffsetUnits=deg  RotationMethod=AlignedAxes  RotationAngleUnits=deg  RotationStandardAxis=+Z  RotationAngle=0.0  RotationArbitraryAxis=[0 0 1]  FollAlignAxisA=+X  BaseAlignAxisA=+Y  FollAlignAxisB=+Y  BaseAlignAxisB=+Z  RotationSequenceAxes=FollowerAxes  RotationSequence=XYX  RotationSequenceAngles=[0 0 0]  RotationSequenceAnglesUnits=deg  RotationMatrix=[1 0 0; 0 1 0; 0 0 1]
  Mechanism Configuration : sm_lib/Utilities/Mechanism Configuration  UniformGravity=Constant  GravityVector=[0 0 -g ]  GravityUnits=m/s^2  LinearizationDelta=1e-4
  PS-Simulink Converter : nesl_utility/PS-Simulink Converter  PhysicalDomain=network_engine_domain  SubClassName=ps_output  LeftPortType=input  RightPortType=output  PseudoPeriodic=off  Frequencies=[]  Unit=rad  AffineConversion=off
  PS-Simulink Converter1 : nesl_utility/PS-Simulink Converter  PhysicalDomain=network_engine_domain  SubClassName=ps_output  LeftPortType=input  RightPortType=output  PseudoPeriodic=off  Frequencies=[]  Unit=rad/s  AffineConversion=off
  PS-Simulink Converter10 : nesl_utility/PS-Simulink Converter  PhysicalDomain=network_engine_domain  SubClassName=ps_output  LeftPortType=input  RightPortType=output  PseudoPeriodic=off  Frequencies=[]  Unit=rad/s  AffineConversion=off
  PS-Simulink Converter11 : nesl_utility/PS-Simulink Converter  PhysicalDomain=network_engine_domain  SubClassName=ps_output  LeftPortType=input  RightPortType=output  PseudoPeriodic=off  Frequencies=[]  Unit=rad/s^2  AffineConversion=off
  PS-Simulink Converter2 : nesl_utility/PS-Simulink Converter  PhysicalDomain=network_engine_domain  SubClassName=ps_output  LeftPortType=input  RightPortType=output  PseudoPeriodic=off  Frequencies=[]  Unit=rad/s^2  AffineConversion=off
  PS-Simulink Converter9 : nesl_utility/PS-Simulink Converter  PhysicalDomain=network_engine_domain  SubClassName=ps_output  LeftPortType=input  RightPortType=output  PseudoPeriodic=off  Frequencies=[]  Unit=rad  AffineConversion=off
  RJ_TH1 : sm_lib/Joints/Revolute Joint  SenseConstraintForce=off  SenseConstraintForceX=off  SenseConstraintForceY=off  SenseConstraintForceZ=off  SenseConstraintTorque=off  SenseConstraintTorqueX=off  SenseConstraintTorqueY=off  SenseConstraintTorqueZ=off  SenseTotalForce=off  SenseTotalForceX=off  SenseTotalForceY=off  SenseTotalForceZ=off  SenseTotalTorque=off  SenseTotalTorqueX=off  SenseTotalTorqueY=off  SenseTotalTorqueZ=off  CompositeWrenchDir=BaseOnFollower  CompositeWrenchFrame=BaseFrame  EquilibriumPosition=0  EquilibriumPositionUnits=deg  SpringStiffness=0  SpringStiffnessUnits=N*m/deg  DampingCoefficient=b1_damp  DampingCoefficientUnits=N*m/(rad/s)  TorqueActuationMode=InputTorque  MotionActuationMode=ComputedMotion  SensePosition=on  SenseVelocity=on  SenseAcceleration=on  SenseTorqueForce=off  PositionTargetSpecify=on  PositionTargetPriority=Low  PositionTargetValue=theta1_0  PositionTargetValueUnits=rad  VelocityTargetSpecify=on  VelocityTargetPriority=High  VelocityTargetValue=theta1_dot_0  VelocityTargetValueUnits=rad/s
      settings: AttributesFormatString=|
      | %<DampingCoefficient>
      | %<PositionTargetValue>
      | %<VelocityTargetValue>
  RJ_TH4_TURN : sm_lib/Joints/Revolute Joint  SenseConstraintForce=off  SenseConstraintForceX=off  SenseConstraintForceY=off  SenseConstraintForceZ=off  SenseConstraintTorque=off  SenseConstraintTorqueX=off  SenseConstraintTorqueY=off  SenseConstraintTorqueZ=off  SenseTotalForce=off  SenseTotalForceX=off  SenseTotalForceY=off  SenseTotalForceZ=off  SenseTotalTorque=off  SenseTotalTorqueX=off  SenseTotalTorqueY=off  SenseTotalTorqueZ=off  CompositeWrenchDir=BaseOnFollower  CompositeWrenchFrame=BaseFrame  EquilibriumPosition=0  EquilibriumPositionUnits=deg  SpringStiffness=0  SpringStiffnessUnits=N*m/deg  DampingCoefficient=b4_damp  DampingCoefficientUnits=N*m/(rad/s)  TorqueActuationMode=InputTorque  MotionActuationMode=ComputedMotion  SensePosition=on  SenseVelocity=on  SenseAcceleration=on  SenseTorqueForce=off  PositionTargetSpecify=on  PositionTargetPriority=Low  PositionTargetValue=theta4_0  PositionTargetValueUnits=rad  VelocityTargetSpecify=on  VelocityTargetPriority=High  VelocityTargetValue=theta4_dot_0  VelocityTargetValueUnits=rad/s
      settings: AttributesFormatString=|
      | %<DampingCoefficient>
      | %<PositionTargetValue>
      | %<VelocityTargetValue>
  RZ2LOCY : sm_lib/Frames and Transforms/Rigid Transform  TranslationMethod=None  TranslationStandardOffset=Hz/2  TranslationLengthUnit=m  TranslationStandardAxis=+Z  TranslationCartesianOffset=[0 0 0]  TranslationROffset=0  TranslationROffsetUnits=m  TranslationZOffset=0  TranslationZOffsetUnits=m  TranslationThetaOffset=0  TranslationThetaOffsetUnits=deg  RotationMethod=AlignedAxes  RotationAngleUnits=deg  RotationStandardAxis=+Z  RotationAngle=0.0  RotationArbitraryAxis=[0 0 1]  FollAlignAxisA=+Y  BaseAlignAxisA=+X  FollAlignAxisB=+X  BaseAlignAxisB=+Z  RotationSequenceAxes=FollowerAxes  RotationSequence=XYX  RotationSequenceAngles=[0 0 0]  RotationSequenceAnglesUnits=deg  RotationMatrix=[1 0 0; 0 1 0; 0 0 1]
  Rigid Transform : sm_lib/Frames and Transforms/Rigid Transform  TranslationMethod=StandardAxis  TranslationStandardOffset=L1y/2  TranslationLengthUnit=m  TranslationStandardAxis=+Y  TranslationCartesianOffset=[0 0 0]  TranslationROffset=0  TranslationROffsetUnits=m  TranslationZOffset=0  TranslationZOffsetUnits=m  TranslationThetaOffset=0  TranslationThetaOffsetUnits=deg  RotationMethod=None  RotationAngleUnits=deg  RotationStandardAxis=+Z  RotationAngle=0.0  RotationArbitraryAxis=[0 0 1]  FollAlignAxisA=+X  BaseAlignAxisA=+Y  FollAlignAxisB=+Y  BaseAlignAxisB=+Z  RotationSequenceAxes=FollowerAxes  RotationSequence=XYX  RotationSequenceAngles=[0 0 0]  RotationSequenceAnglesUnits=deg  RotationMatrix=[1 0 0; 0 1 0; 0 0 1]
  Rigid Transform1 : sm_lib/Frames and Transforms/Rigid Transform  TranslationMethod=StandardAxis  TranslationStandardOffset=L1y/2  TranslationLengthUnit=m  TranslationStandardAxis=+Y  TranslationCartesianOffset=[0 0 0]  TranslationROffset=0  TranslationROffsetUnits=m  TranslationZOffset=0  TranslationZOffsetUnits=m  TranslationThetaOffset=0  TranslationThetaOffsetUnits=deg  RotationMethod=None  RotationAngleUnits=deg  RotationStandardAxis=+Z  RotationAngle=0.0  RotationArbitraryAxis=[0 0 1]  FollAlignAxisA=+X  BaseAlignAxisA=+Y  FollAlignAxisB=+Y  BaseAlignAxisB=+Z  RotationSequenceAxes=FollowerAxes  RotationSequence=XYX  RotationSequenceAngles=[0 0 0]  RotationSequenceAnglesUnits=deg  RotationMatrix=[1 0 0; 0 1 0; 0 0 1]
  Rigid Transform5 : sm_lib/Frames and Transforms/Rigid Transform  TranslationMethod=StandardAxis  TranslationStandardOffset=Hz/2  TranslationLengthUnit=m  TranslationStandardAxis=-Z  TranslationCartesianOffset=[0 0 0]  TranslationROffset=0  TranslationROffsetUnits=m  TranslationZOffset=0  TranslationZOffsetUnits=m  TranslationThetaOffset=0  TranslationThetaOffsetUnits=deg  RotationMethod=None  RotationAngleUnits=deg  RotationStandardAxis=+Z  RotationAngle=0.0  RotationArbitraryAxis=[0 0 1]  FollAlignAxisA=+X  BaseAlignAxisA=+Y  FollAlignAxisB=+Y  BaseAlignAxisB=+Z  RotationSequenceAxes=FollowerAxes  RotationSequence=XYX  RotationSequenceAngles=[0 0 0]  RotationSequenceAnglesUnits=deg  RotationMatrix=[1 0 0; 0 1 0; 0 0 1]
  Rigid Transform6 : sm_lib/Frames and Transforms/Rigid Transform  TranslationMethod=StandardAxis  TranslationStandardOffset=Hz/2  TranslationLengthUnit=m  TranslationStandardAxis=+Z  TranslationCartesianOffset=[0 0 0]  TranslationROffset=0  TranslationROffsetUnits=m  TranslationZOffset=0  TranslationZOffsetUnits=m  TranslationThetaOffset=0  TranslationThetaOffsetUnits=deg  RotationMethod=None  RotationAngleUnits=deg  RotationStandardAxis=+Z  RotationAngle=0.0  RotationArbitraryAxis=[0 0 1]  FollAlignAxisA=+X  BaseAlignAxisA=+Y  FollAlignAxisB=+Y  BaseAlignAxisB=+Z  RotationSequenceAxes=FollowerAxes  RotationSequence=XYX  RotationSequenceAngles=[0 0 0]  RotationSequenceAnglesUnits=deg  RotationMatrix=[1 0 0; 0 1 0; 0 0 1]
  Solver Configuration : nesl_utility/Solver Configuration  PhysicalDomain=network_engine_domain  SubClassName=solver  LeftPortType=input  RightPortType=generic  Accelerate=off  Tones=[]  Harmonics=[]  SimulateNoise=off  Profile=off  UseLocalSampling=off  EnableSwitchedLinearOptims=on  FrequencyDomain=off  UseCCode=off  RelTol=0.001  AbsTol=1e-06  MinStep=1e-09  ToWorkspace=off  RevertToSquareIcSolve=off  NumHomotopyIterations=100  PhasorMode=off  PhasorModeNumHarmonics=1  OverrideAbsTol=off  DoDC=off  ResidualTolerance=1e-09  UseLocalSolver=off  LocalSolverChoice=NE_TRAPEZOIDAL_ADVANCER  LocalSolverSampleTime=0.01  DoFixedCost=off  MaxNonlinIter=3  MaxModeIter=2  LinearAlgebra=Sparse  DelaysMemoryBudget=1024  AutomaticFiltering=on  FilteringTimeConstant=0.001
  TURNTABLE : sm_lib/Body Elements/Solid  InertiaType=CalculateFromGeometry  Mass=1  MassUnits=kg  CenterOfMass=[0 0 0]  CenterOfMassUnits=m  MomentsOfInertia=[1 1 1]  MomentsOfInertiaUnits=kg*m^2  ProductsOfInertia=[0 0 0]  ProductsOfInertiaUnits=kg*m^2  DensityBased=on  Density=density  DensityUnits=kg/(m^3)  DoExposeReferenceFrame=on  SerializedFrames=<Frames/>  GraphicType=FromGeometry  MarkerShape=Sphere  MarkerSize=10  GraphicVisPropType=SimpleVisualProperties  GraphicDiffuseColor=[1.0 1.0 0.2]  GraphicSpecularColor=[0.5 0.5 0.5 1.0]  GraphicAmbientColor=[0.15 0.15 0.15 1.0]  GraphicEmissiveColor=[0.0 0.0 0.0 1.0]  GraphicShininess=75  GraphicOpacity=1.0  GeometryShape=Cylinder  RectangleSize=[1 1]  RectangleSizeUnits=m  BrickDimensions=[1 1 1]  BrickDimensionUnits=m  CylinderRadius=Rturn  CylinderRadiusUnits=m  CylinderLength=Hz  CylinderLengthUnits=m  SphereRadius=1  SphereRadiusUnits=m  EllipsoidRadii=[1 1 1]  EllipsoidRadiiUnits=m  ExtrusionCrossSection=[1 1; -1 1; -1 -1; 1 -1]  ExtrusionCrossSectionUnits=m  ExtrusionLength=1  ExtrusionLengthUnits=m  PolygonNumSides=3  PolygonOuterRadius=1  PolygonOuterRadiusUnits=m  ExtGeomFileType=STEP  ExtGeomFileUnits=m  RevolutionCrossSection=[1 1; 1 -1; 2 -1; 2 1]  RevolutionCrossSectionUnits=m  RevolutionExtent=Full  RevolutionAngle=180  RevolutionAngleUnits=deg
  World Frame : sm_lib/Frames and Transforms/World Frame
  TQ1 : PMIOPort  Port=1  Side=Left
  W1 : PMIOPort  Port=2  Side=Left
  TQ4 : PMIOPort  Port=3  Side=Left
  W4 : PMIOPort  Port=4  Side=Left
  TH1 : Outport
  TH1_D : Outport  Port=2
  TH1_DD : Outport  Port=3
  TH4 : Outport  Port=4
  TH4_D : Outport  Port=5
  TH4_DD : Outport  Port=6
  wires:
  PS-Simulink Converter/1 -> [TH1]  "TH1"
  PS-Simulink Converter2/1 -> [TH1_DD]  "TH1_DD"
  PS-Simulink Converter1/1 -> [TH1_D]  "TH1_D"
  PS-Simulink Converter9/1 -> [TH4]  "TH4"
  PS-Simulink Converter11/1 -> [TH4_DD]  "TH4_DD"
  PS-Simulink Converter10/1 -> [TH4_D]  "TH4_D"
  [TH1] -> TH1/1
  [TH1_D] -> TH1_D/1
  [TH1_DD] -> TH1_DD/1
  [TH4_DD] -> TH4_DD/1
  [TH4_D] -> TH4_D/1
  [TH4] -> TH4/1
  connections:
  Mechanism Configuration/RConn1 -- RJ_TH4_TURN/LConn1 -- Solver Configuration/RConn1 -- World Frame/RConn1
  Rigid Transform6/LConn1 -- TURNTABLE/RConn1 -- Rigid Transform5/RConn1
  LINK_1/RConn1 -- Rigid Transform/RConn1 -- Rigid Transform1/LConn1
  TQ1/RConn1 -- RJ_TH1/LConn2
  RZ2LOCY/RConn1 -- Rigid Transform/LConn1
  RJ_TH4_TURN/RConn3 -- W4/RConn1 -- PS-Simulink Converter10/LConn1
  PS-Simulink Converter1/LConn1 -- W1/RConn1 -- RJ_TH1/RConn3
  LocY2RZ/LConn1 -- Rigid Transform6/RConn1
  Rigid Transform5/LConn1 -- RJ_TH4_TURN/RConn1
  LocY2RZ/RConn1 -- RJ_TH1/LConn1
  LocY2RZ2/LConn1 -- Rigid Transform1/RConn1
  PS-Simulink Converter2/LConn1 -- RJ_TH1/RConn4
  RJ_TH1/RConn1 -- RZ2LOCY/LConn1
  RJ_TH4_TURN/RConn4 -- PS-Simulink Converter11/LConn1
  RJ_TH4_TURN/RConn2 -- PS-Simulink Converter9/LConn1
  PS-Simulink Converter/LConn1 -- RJ_TH1/RConn2
  TQ4/RConn1 -- RJ_TH4_TURN/LConn2

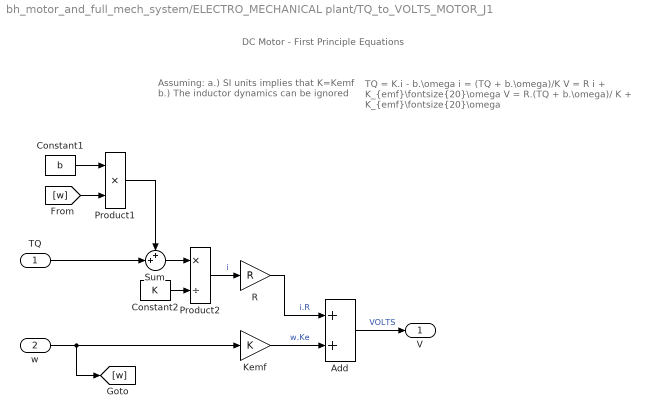
== system bh_motor_and_full_mech_system/ELECTRO_MECHANICAL plant/TQ_to_VOLTS_MOTOR_J1 ==
  note: TQ = K.i  - b.\omega
      |
      | i = (TQ + b.\omega)/K
      |
      | V = R i   +   K_{emf}\fontsize{20}\omega
      |
      | V = R.(TQ  + b.\omega)/ K   +    K_{emf}\fontsize{20}\omega
  note: DC Motor - First Principle Equations
  note: Assuming:
      |  a.) SI units implies that   K=Kemf
      |  b.) The inductor dynamics can be ignored
  TQ : Inport
  w : Inport  Port=2
  Add : Sum
  Constant1 : Constant  Value=b
  Constant2 : Constant  Value=K
  Kemf : Gain  Gain=K
  Product1 : Product
  Product2 : Product  Inputs=*/
  R : Gain  Gain=R
  Sum : Sum  Inputs=++|
  V : Outport
  wires:
  R/1 -> Add/1  "i.R"
  Product2/1 -> R/1  "i"
  Constant2/1 -> Product2/2
  Kemf/1 -> Add/2  "w.Ke"
  w/1 -> [w], Kemf/1
  Add/1 -> V/1  "VOLTS"
  Sum/1 -> Product2/1
  TQ/1 -> Sum/2
  Constant1/1 -> Product1/1
  [w] -> Product1/2
  Product1/1 -> Sum/1

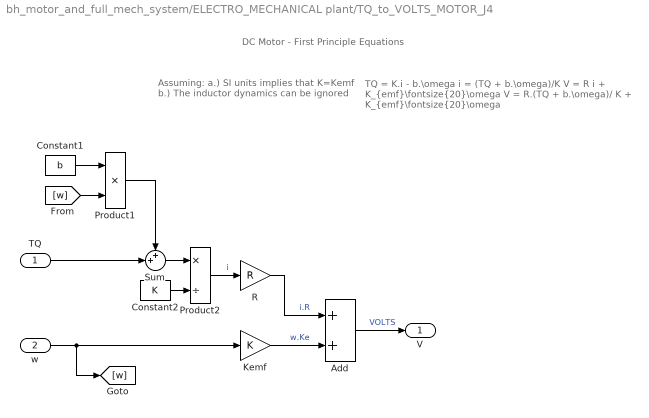
== system bh_motor_and_full_mech_system/ELECTRO_MECHANICAL plant/TQ_to_VOLTS_MOTOR_J4 ==
  note: TQ = K.i  - b.\omega
      |
      | i = (TQ + b.\omega)/K
      |
      | V = R i   +   K_{emf}\fontsize{20}\omega
      |
      | V = R.(TQ  + b.\omega)/ K   +    K_{emf}\fontsize{20}\omega
  note: DC Motor - First Principle Equations
  note: Assuming:
      |  a.) SI units implies that   K=Kemf
      |  b.) The inductor dynamics can be ignored
  TQ : Inport
  w : Inport  Port=2
  Add : Sum
  Constant1 : Constant  Value=b
  Constant2 : Constant  Value=K
  Kemf : Gain  Gain=K
  Product1 : Product
  Product2 : Product  Inputs=*/
  R : Gain  Gain=R
  Sum : Sum  Inputs=++|
  V : Outport
  wires:
  R/1 -> Add/1  "i.R"
  Product2/1 -> R/1  "i"
  Constant2/1 -> Product2/2
  Kemf/1 -> Add/2  "w.Ke"
  w/1 -> [w], Kemf/1
  Add/1 -> V/1  "VOLTS"
  Sum/1 -> Product2/1
  TQ/1 -> Sum/2
  Constant1/1 -> Product1/1
  [w] -> Product1/2
  Product1/1 -> Sum/1

== system bh_motor_and_full_mech_system/ELECTRO_MECHANICAL plant/interface 1D_to_3D ==
  Ideal Angular Velocity Source : fl_lib/Mechanical/Mechanical Sources/Ideal Angular Velocity Source
  Ideal Torque Sensor2 : fl_lib/Mechanical/Mechanical Sensors/Ideal Torque Sensor
  SHAFT : PMIOPort  Port=1  Side=Left
  mech_REF : PMIOPort  Port=2  Side=Left
  TQ : PMIOPort  Port=3  Side=Right
  w : PMIOPort  Port=4  Side=Right
  connections:
  Ideal Torque Sensor2/RConn2 -- TQ/RConn1
  Ideal Angular Velocity Source/RConn1 -- w/RConn1
  Ideal Angular Velocity Source/LConn1 -- Ideal Torque Sensor2/RConn1
  SHAFT/RConn1 -- Ideal Torque Sensor2/LConn1
  mech_REF/RConn1 -- Ideal Angular Velocity Source/RConn2

== system bh_motor_and_full_mech_system/ELECTRO_MECHANICAL plant/interface 1D_to_3D1 ==
  Ideal Angular Velocity Source : fl_lib/Mechanical/Mechanical Sources/Ideal Angular Velocity Source
  Ideal Torque Sensor2 : fl_lib/Mechanical/Mechanical Sensors/Ideal Torque Sensor
  SHAFT : PMIOPort  Port=1  Side=Left
  mech_REF : PMIOPort  Port=2  Side=Left
  TQ : PMIOPort  Port=3  Side=Right
  w : PMIOPort  Port=4  Side=Right
  connections:
  Ideal Torque Sensor2/RConn2 -- TQ/RConn1
  Ideal Angular Velocity Source/RConn1 -- w/RConn1
  Ideal Angular Velocity Source/LConn1 -- Ideal Torque Sensor2/RConn1
  SHAFT/RConn1 -- Ideal Torque Sensor2/LConn1
  mech_REF/RConn1 -- Ideal Angular Velocity Source/RConn2
